simulink model "CONTROL_01"  (R2018b)
settings: Solver=FixedStepAuto  StartTime=0.0  StopTime=30  FixedStep=0.01  RelTol=1e-3
model workspace: external: MATLAB File D:\OneDrive\STUDY\RIC LAB\PROJECT 6DOF\CODE\CODE 6DOF\07_CONTROL\CONTROL_02\ROBOT_DataFile.m (data not in the file)
undefined symbols (not defined in the file or in its folder): smiData, X, Y, Z
libraries: sm_lib x35, nesl_utility x7
(part 124 of 185)

== matlab function CONTROL_01/PID Control/PID ==
  data: e input; ei input; to output; ed input; Kp input; Ki input; Kd input
function to = fcn(e,ei,ed,Kp,Ki,Kd)
Kp_ = diag(Kp);
Ki_ = diag(Ki);
Kd_ = diag(Kd);
to = Kp_*e + Ki_*ei + Kd_*ed;
